simulink model "power_upfc"  (Simulink 8.3)
settings: Solver=ode23tb  SolverMode=SingleTasking  StartTime=0  StopTime=20  MaxStep=1/60  RelTol=1e-4  AbsTol=1e-3
undefined symbols (not defined in the file or in its folder): D1, Delta
libraries: powerlib x30, powerlib_meascontrol x12, sps_avr x2, factslib x1, simulink x1
Description:
  | Copyright 2008-2014 The MathWorks, Inc.
settings Model: Creator=MathWorks  LastModifiedBy=snt  ExtModeAutoUpdateStatusClock=off
settings SolverCC: SolverJacobianMethodControl=FullPerturbation
settings DataIOCC: LimitDataPoints=off  SaveOutput=off  SaveTime=off  SignalLoggingName=sigsOut
settings OptimizationCC: BooleanDataType=off  ExpressionDepthLimit=2147483647  InitFltsAndDblsToZero=on  EfficientMapNaN2IntZero=off
settings DebuggingCC: CheckExecutionContextPreStartOutputMsg=on  CheckExecutionContextRuntimeOutputMsg=on  SignalResolutionControl=TryResolveAllWithWarning  SolverPrmCheckMsg=none  MultiTaskDSMMsg=warning  MultiTaskCondExecSysMsg=none  SigSpecEnsureSampleTimeMsg=none  FcnCallInpInsideContextMsg=UseLocalSettings  UnconnectedInputMsg=none  UnconnectedOutputMsg=none  UnconnectedLineMsg=none
settings HardwareCC: TargetUnknown=on
settings RTWCC: IncludeERTFirstTime=on
settings CodeAppCC: IgnoreCustomStorageClasses=off

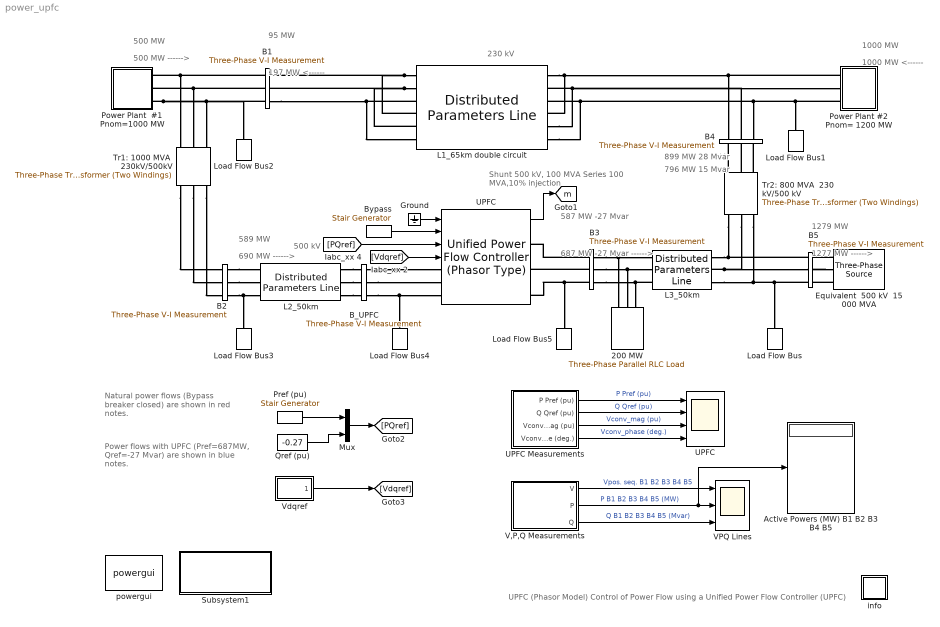
== system power_upfc ==
  note: Shunt 500 kV, 100 MVA
      | Series 100 MVA,10% injection
  note: 1000 MW
      | <------
  note: I
      | I
      | V
  note: 197 MW
      | <------
  note: 1277 MW
      | ------>
  note: 500 MW
      | ------>
  note: 690 MW
      | ------>
  note: 687 MW -27 Mvar
      |           ------>
  note: 230 kV
  note: 500 kV
  note: UPFC (Phasor Model)
      | Control of Power Flow using a Unified Power Flow Controller (UPFC)
  note: 796 MW 15 Mvar
  note: 95 MW
  note: 500 MW
  note: 1000 MW
  note: 589 MW
  note: 587 MW -27 Mvar
  note: 1279 MW
  note: 899 MW 28 Mvar
  note: Natural power flows
      | (Bypass breaker closed)
      | are shown in red notes.
  note: Power flows with UPFC
      | (Pref=687MW, Qref=-27 Mvar)
      | are shown in blue notes.
  200 MW : powerlib/Elements/Three-Phase Parallel RLC Load  LConnTagsString=A|B|C  Configuration=Y (grounded)  NominalVoltage=500e3  NominalFrequency=60  ActivePower=2e+008  InductivePower=0  CapacitivePower=0  Measurements=None  LoadType=constant Z
  Active Powers (MW) B1 B2 B3 B4 B5 : Display
      settings: SampleTime=0.1
  B1 : powerlib/Measurements/Three-Phase V-I Measurement  VoltageMeasurement=phase-to-ground  SetLabelV=on  LabelV=Vabc_B1  Vpu=on  VpuLL=off  CurrentMeasurement=yes  SetLabelI=on  LabelI=Iabc_B1  Ipu=on  Pbase=100e6  Vbase=230e3  OutputType=Complex  PhasorSimulation=on  PSBequivalent=0
  B2 : powerlib/Measurements/Three-Phase V-I Measurement  VoltageMeasurement=phase-to-ground  SetLabelV=on  LabelV=Vabc_B2  Vpu=on  VpuLL=off  CurrentMeasurement=yes  SetLabelI=on  LabelI=Iabc_B2  Ipu=on  Pbase=100e6  Vbase=500e3  OutputType=Complex  PhasorSimulation=on  PSBequivalent=0
  B3 : powerlib/Measurements/Three-Phase V-I Measurement  VoltageMeasurement=phase-to-ground  SetLabelV=on  LabelV=Vabc_B3  Vpu=on  VpuLL=off  CurrentMeasurement=yes  SetLabelI=on  LabelI=Iabc_B3  Ipu=on  Pbase=100e6  Vbase=500e3  OutputType=Complex  PhasorSimulation=on  PSBequivalent=0
  B4 : powerlib/Measurements/Three-Phase V-I Measurement  VoltageMeasurement=phase-to-ground  SetLabelV=on  LabelV=Vabc_B4  Vpu=on  VpuLL=off  CurrentMeasurement=yes  SetLabelI=on  LabelI=Iabc_B4  Ipu=on  Pbase=100e6  Vbase=230e3  OutputType=Complex  PhasorSimulation=on  PSBequivalent=0
  B5 : powerlib/Measurements/Three-Phase V-I Measurement  VoltageMeasurement=phase-to-ground  SetLabelV=on  LabelV=Vabc_B5  Vpu=on  VpuLL=off  CurrentMeasurement=yes  SetLabelI=on  LabelI=Iabc_B5  Ipu=on  Pbase=100e6  Vbase=500e3  OutputType=Complex  PhasorSimulation=on  PSBequivalent=0
  B_UPFC : powerlib/Measurements/Three-Phase V-I Measurement  VoltageMeasurement=phase-to-ground  SetLabelV=on  LabelV=Vabc_UPFC  Vpu=on  VpuLL=off  CurrentMeasurement=no  SetLabelI=on  LabelI=Iabc_UPFC  Ipu=on  Pbase=100e6  Vbase=500e3  OutputType=Complex  PhasorSimulation=on  PSBequivalent=0
  Bypass : powerlib_meascontrol/Pulse & Signal Generators/Stair Generator  t=[0,5]  e=[1, 0]  Ts=0
  Equivalent  500 kV  15 000 MVA : powerlib/Electrical Sources/Three-Phase Source  Voltage=(500000)*1  PhaseAngle=3.2028e-005  Frequency=60  InternalConnection=Yg  SpecifyImpedance=on  Resistance=0.8929  Inductance=16.58e-3  ShortCircuitLevel=15000e6  BaseVoltage=500e3  XRratio=10  BusType=swing  Pref=0  Qref=0  Qmin=-Inf  Qmax=Inf
  Ground : Ground
  L1_65km double circuit : powerlib/Elements/Distributed Parameters Line  Phases=6  Frequency=60  Resistance="[0.068  0.284  0.216]"  Inductance="[1.31e-3  4.02e-3  2.43e-3]"  Capacitance="[8.85e-9  6.21e-9  -1.88e-9]"  Length=65  x1=[1.04987199469285e-07 0 229205.80796604 229205.606293905 229205.80796604 229205.606293905;376.991118430775 376.991118430775 376.991118430775 376.991118430775 376.991118430775 376.991118430775;1.60854183298652 0 0.666699049272692 -0.904097686354923 0.666699049272692 -0.904097686354923]  x2=[6.52522329341896e-07 7.27595761418343e-12 228285.721081789 228285.608536952 228285.721081789 228285.608536952;376.991118430775 376.991118430775 376.991118430775 376.991118430775 376.991118430775 376.991118430775;1.99334329783026 -0.0878855142633377 0.697028223829494 -0.873768326941681 0.697028223829494 -0.873768326941681]  x3=[3.46977339890718e-09 9.30248222866475e-13 797.813028086103 797.813944366895 797.813028086104 797.813944366895;376.991118430775 376.991118430775 376.991118430775 376.991118430775 376.991118430775 376.991118430775;0.713863028790556 0.253093439233012 0.71113154759669 -0.859668364592689 0.71113154759669 -0.859668364592689]  x4=[3.27711624608603e-09 8.10443810681981e-13 388.164983704915 388.162721923639 388.164983704915 388.16272192364;376.991118430775 376.991118430775 376.991118430775 376.991118430775 376.991118430775 376.991118430775;-2.59754346741824 0.0169914244668962 0.493384723437739 -1.07740616674268 0.493384723437737 -1.07740616674268]  x5=0.000343508242259192  V1=ones(3,3)  V2=ones(3,3)  I1=ones(3,3)  I2=ones(3,3)  nHarmo=1  Measurements=None
      settings: AttributesFormatString=\n
  L2_50km : powerlib/Elements/Distributed Parameters Line  Phases=3  Frequency=60  Resistance=[0.01273*2 0.3864]  Inductance="[0.9337e-3  4.1264e-3]"  Capacitance=[12.74e-9 7.751e-9]  Length=50  x1=[5.20853276713395e-08 499627.087562911 499626.799727799;376.991118430775 376.991118430775 376.991118430775;1.55035171690532 0.613862513789087 -0.956934116072279]  x2=[4.53565246682871e-08 499734.367587277 499734.166072354;376.991118430775 376.991118430775 376.991118430775;0.508276734166516 0.572208220004921 -0.998588334903276]  x3=[5.37095681221166e-10 675.32888932722 675.331629163871;376.991118430775 376.991118430775 376.991118430775;-2.03735480978532 0.425693420201668 -1.14510959351009]  x4=[6.51364168678501e-10 3011.82389463488 3011.82010569616;376.991118430775 376.991118430775 376.991118430775;1.09280353932366 0.590627024477705 -0.980167982447582]  x5=0.000282770783497871  V1=ones(3,3)  V2=ones(3,3)  I1=ones(3,3)  I2=ones(3,3)  nHarmo=1  Measurements=None
      settings: AttributesFormatString=\n
  L3_50km : powerlib/Elements/Distributed Parameters Line  Phases=3  Frequency=60  Resistance=[0.01273*2 0.3864]  Inductance="[0.9337e-3  4.1264e-3]"  Capacitance=[12.74e-9 7.751e-9]  Length=50  x1=[4.54922196369805e-08 499734.250125523 499734.048610914;376.991118430775 376.991118430775 376.991118430775;0.506954071581508 0.572208208878681 -0.998588346030441]  x2=[7.60694684117164e-08 498857.669479026 498857.551895537;376.991118430775 376.991118430775 376.991118430775;-0.0702475012256047 0.544899092106288 -1.02589737598285]  x3=[5.13234018676451e-10 1067.88465961171 1067.8871249624;376.991118430775 376.991118430775 376.991118430775;-1.90562270617231 0.520240004579847 -1.0505607358324]  x4=[5.95962577824804e-10 2609.42085232127 2609.41725096603;376.991118430775 376.991118430775 376.991118430775;0.999199616559189 0.528387817683497 -1.04240695612209]  x5=0.000282770783497871  V1=ones(3,3)  V2=ones(3,3)  I1=ones(3,3)  I2=ones(3,3)  nHarmo=1  Measurements=None
      settings: AttributesFormatString=\n
  Load Flow Bus : powerlib/Measurements/Load Flow Bus  LConnTagsString=a  ID=B5  Vbase=500e3  Vref=0.997715  Vangle=4.9453  VLF=0.9977  angleLF=4.945
      settings: AttributesFormatString=%<ID>\n%<Vbase>V\n%<VLF>pu\n%<angleLF>deg.
  Load Flow Bus1 : powerlib/Measurements/Load Flow Bus  LConnTagsString=a  ID=B4  Vbase=230e3  Vref=1  Vangle=0  VLF=0.9925  angleLF=14.72
      settings: AttributesFormatString=%<ID>\n%<Vbase>V\n%<VLF>pu\n%<angleLF>deg.
  Load Flow Bus2 : powerlib/Measurements/Load Flow Bus  LConnTagsString=a  ID=B1  Vbase=230e3  Vref=1  Vangle=0  VLF=0.9965  angleLF=12.98
      settings: AttributesFormatString=%<ID>\n%<Vbase>V\n%<VLF>pu\n%<angleLF>deg.
  Load Flow Bus3 : powerlib/Measurements/Load Flow Bus  LConnTagsString=a  ID=B2  Vbase=500e3  Vref=1  Vangle=0  VLF=0.9993  angleLF=8.897
      settings: AttributesFormatString=%<ID>\n%<Vbase>V\n%<VLF>pu\n%<angleLF>deg.
  Load Flow Bus4 : powerlib/Measurements/Load Flow Bus  LConnTagsString=a  ID=B_UPFC  Vbase=500e3  Vref=1  Vangle=0  VLF=0.9995  angleLF=6.51
      settings: AttributesFormatString=%<ID>\n%<Vbase>V\n%<VLF>pu\n%<angleLF>deg.
  Load Flow Bus5 : powerlib/Measurements/Load Flow Bus  LConnTagsString=a  ID=B3  Vbase=500e3  Vref=1  Vangle=0  VLF=0.9995  angleLF=6.51
      settings: AttributesFormatString=%<ID>\n%<Vbase>V\n%<VLF>pu\n%<angleLF>deg.
  Mux : Mux  Inputs=2
  Power Plant  #1 Pnom=1000 MW : Subsystem
  Power Plant #2 Pnom= 1200 MW : Subsystem
  Pref (pu) : powerlib_meascontrol/Pulse & Signal Generators/Stair Generator  t=[0,10]  e="[5.87 6.87  ]"  Ts=0
  Qref (pu) : Constant  Value=-0.27
  Subsystem1 : Subsystem
      settings: OpenFcn=|
      | if exist('P_SE') & exist('Q_SE')
      | plot(P_SE(300:length(Q_SE),2),Q_SE(300:length(Q_SE),2))
      | pbaspect([1 1 1]);
      |    grid
      | title('UPFC Controllable Region')
      | xlabel ('P (pu)')
      | ylabel ('Q (pu)')
      | end
      mask Display: disp('Double click to plot\nUPFC\nControllable Region')
  Tr1: 1000 MVA  230kV/500kV : powerlib/Elements/Three-Phase Transformer (Two Windings)  Winding1Connection=Yg  UNITS=pu  NominalPower=[ 1000e6 60 ]  Winding1="[ 230e3 0.002  0.0]"  Winding2Connection=Yg  Winding2=[ 500e3 0.002 0.12]  SetSaturation=off  Rm=500  Lm=500  Saturation="[ 0,0  ;  0.005,1.2  ;  1.0,1.4 ]"  Hysteresis=off  DataFile='basic_model'  SetInitialFlux=off  InitialFluxes=[ 0.8 , -0.8 , 0.7 ]  Measurements=None  MoreParameters=off  BreakLoop=off  DataType=off  TransfoNumber=0
  Tr2: 800 MVA  230 kV/500 kV : powerlib/Elements/Three-Phase Transformer (Two Windings)  Winding1Connection=Yg  UNITS=pu  NominalPower=[ 800e6 60 ]  Winding1="[ 230e3 0.002  0.0]"  Winding2Connection=Yg  Winding2=[ 500e3 0.002 0.15]  SetSaturation=off  Rm=500  Lm=500  Saturation="[ 0,0  ;  0.005,1.2  ;  1.0,1.4 ]"  Hysteresis=off  DataFile='basic_model'  SetInitialFlux=off  InitialFluxes=[ 0.8 , -0.8 , 0.7 ]  Measurements=None  MoreParameters=off  BreakLoop=off  DataType=off  TransfoNumber=0
  UPFC : factslib/Power-Electronics Based FACTS/Unified Power Flow Controller (Phasor Type)  ShowParameters=Control parameters (series converter)  SystemNominal=[ 500e3, 60 ]  Pnom_SH=100e6  RL_SH=[ 0.22/30, 0.22 ]  Iinit_SH=[0, 0 ]  SeriesNominal=[ 100e6, 0.1]  RL_SE=[ 0.16/30, 0.16 ]  Iinit_SE=[ 0 0]  VnomDC=40000  C_DC=750e-6  OpMode_SH=Voltage regulation  ExternalVref=off  Vref_SH=1.00  MaxRateChangeVref_SH=0.1  Droop_SH=0.03  Par_VacReg=[5 1000]  Qref_SH=0  MaxRateChangeQref_SH=2  Par_VdcReg=[0.1e-3 20e-3]  Par_IReg_SH=[0.5 25]/3  ExternalByPass=External control  OpMode_SE=Power flow control  ExternalPQref=on  PQref_SE=[5.87 -0.27]  Rate_PQref=1  Par_PReg_SE=[0.025 1.5]  ExternalVdqref=on  Vdqref_SE=[0.05 0.05]  Rate_Vdqref=0.2
  UPFC Measurements : Subsystem
      mask Display: disp('UPFC\nMeasurements')
  "UPFC " : Scope  NumInputPorts=4
      settings: TimeRange=20  YMin=5.5~-0.29~0~90  YMax=7~-0.26~0.1~96
  V,P,Q Measurements : Subsystem
      mask Display: disp('V P Q\nMeasurements')
  VPQ Lines : Scope  NumInputPorts=3
      settings: TimeRange=20  YMin=0.99~0~-150  YMax=1.005~1500~50
  Vdqref : Subsystem
  info : Subsystem
      settings: OpenFcn=showdemo(bdroot(gcb))
      mask Display: disp('?')
  powergui : powerlib/powergui  Priority=2  SimulationMode=Phasor  SolverType=Tustin  SampleTime=0  frequency=60  SPID=off  DisableSnubberDevices=off  DisableRonSwitches=off  DisableVfSwitches=off  SwTol=0  Interpol=off  DisplayEquations=off  Ts=0  methode=off  frequencyindice=60  Pbase=100e6  ErrMax=0.0001  Iterations=50  UnitsV=kV  UnitsW=MW  FunctionMessages=off  echomessages=off  HookPort=off  EnableUseOfTLC=off  x0status=blocks  RestoreLinks=warning  ResistiveCurrentMeasurement=off  Frange=[0:2:500]  Ylog=off  Xlog=off  ShowGrid=off  save=off  variable=ZData  structure=0  ZoomFFT=on  StartTime=0.0  cycles=1  DisplayStyle=off  fundamental=60  FreqAxis=off  MaxFrequency=1000  frequencyindicesteady=1  RmsSteady=2  display=off
  tag scope: m=global
  wires:
  Pref (pu)/1 -> Mux/1
  Qref (pu)/1 -> Mux/2
  Mux/1 -> [PQref]
  V,P,Q Measurements/1(V) -> VPQ Lines/1  "Vpos. seq. B1 B2 B3 B4 B5"
  UPFC/1 -> [m]
  Vdqref/1(Vdqref) -> [Vdqref]
  V,P,Q Measurements/3(Q) -> VPQ Lines/3  "Q B1 B2 B3 B4 B5 (Mvar)"
  UPFC Measurements/1(P Pref (pu)) -> "UPFC "/1  "P Pref (pu)"
  UPFC Measurements/2(Q Qref (pu)) -> "UPFC "/2  "Q Qref (pu)"
  UPFC Measurements/3(Vconv_mag (pu)) -> "UPFC "/3  "Vconv_mag (pu)"
  UPFC Measurements/4(Vconv_phase (deg.)) -> "UPFC "/4  "Vconv_phase (deg.)"
  V,P,Q Measurements/2(P) -> VPQ Lines/2, Active Powers (MW) B1 B2 B3 B4 B5/1  "P B1 B2 B3 B4 B5 (MW)"
  Ground/1 -> UPFC/1
  [Vdqref] -> UPFC/4
  [PQref] -> UPFC/3
  Bypass/1 -> UPFC/2
  connections:
  Equivalent  500 kV  15 000 MVA/RConn1 -- B5/RConn1
  B5/RConn2 -- Equivalent  500 kV  15 000 MVA/RConn2
  Equivalent  500 kV  15 000 MVA/RConn3 -- B5/RConn3
  Power Plant #2 Pnom= 1200 MW/RConn3 -- L1_65km double circuit/RConn3 -- L1_65km double circuit/RConn6 -- B4/LConn3 -- Load Flow Bus1/LConn1
  L3_50km/RConn1 -- B5/LConn1 -- Tr2: 800 MVA  230 kV/500 kV/RConn1
  L3_50km/RConn2 -- B5/LConn2 -- Tr2: 800 MVA  230 kV/500 kV/RConn2
  B5/LConn3 -- L3_50km/RConn3 -- Tr2: 800 MVA  230 kV/500 kV/RConn3 -- Load Flow Bus/LConn1
  B4/LConn2 -- Power Plant #2 Pnom= 1200 MW/RConn2 -- L1_65km double circuit/RConn2 -- L1_65km double circuit/RConn5
  B3/RConn1 -- L3_50km/LConn1 -- 200 MW/LConn1
  B3/RConn2 -- L3_50km/LConn2 -- 200 MW/LConn2
  B3/RConn3 -- L3_50km/LConn3 -- 200 MW/LConn3
  B2/RConn1 -- L2_50km/LConn1
  B2/RConn2 -- L2_50km/LConn2
  B2/RConn3 -- L2_50km/LConn3 -- Load Flow Bus3/LConn1
  B1/RConn1 -- Power Plant  #1 Pnom=1000 MW/RConn1 -- Tr1: 1000 MVA  230kV/500kV/LConn1
  B1/RConn2 -- Power Plant  #1 Pnom=1000 MW/RConn2 -- Tr1: 1000 MVA  230kV/500kV/LConn2
  Power Plant  #1 Pnom=1000 MW/RConn3 -- B1/RConn3 -- Load Flow Bus2/LConn1 -- Tr1: 1000 MVA  230kV/500kV/LConn3
  Tr1: 1000 MVA  230kV/500kV/RConn1 -- B2/LConn1
  Tr1: 1000 MVA  230kV/500kV/RConn2 -- B2/LConn2
  Tr1: 1000 MVA  230kV/500kV/RConn3 -- B2/LConn3
  Tr2: 800 MVA  230 kV/500 kV/LConn1 -- B4/RConn1
  Tr2: 800 MVA  230 kV/500 kV/LConn2 -- B4/RConn2
  Tr2: 800 MVA  230 kV/500 kV/LConn3 -- B4/RConn3
  L2_50km/RConn1 -- B_UPFC/LConn1
  L2_50km/RConn2 -- B_UPFC/LConn2
  L2_50km/RConn3 -- B_UPFC/LConn3
  B_UPFC/RConn1 -- UPFC/LConn1
  B_UPFC/RConn2 -- UPFC/LConn2
  B_UPFC/RConn3 -- UPFC/LConn3 -- Load Flow Bus4/LConn1
  B3/LConn1 -- UPFC/RConn1
  B3/LConn2 -- UPFC/RConn2
  B3/LConn3 -- UPFC/RConn3 -- Load Flow Bus5/LConn1
  L1_65km double circuit/LConn1 -- B1/LConn1 -- L1_65km double circuit/LConn4
  L1_65km double circuit/LConn2 -- B1/LConn2 -- L1_65km double circuit/LConn5
  B1/LConn3 -- L1_65km double circuit/LConn3 -- L1_65km double circuit/LConn6
  L1_65km double circuit/RConn1 -- Power Plant #2 Pnom= 1200 MW/RConn1 -- B4/LConn1 -- L1_65km double circuit/RConn4

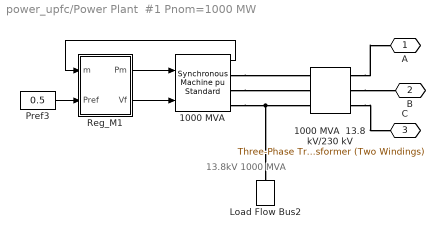
== system power_upfc/Power Plant  #1 Pnom=1000 MW ==
  note: 13.8kV 1000 MVA
  1000 MVA : powerlib/Machines/Synchronous Machine pu Standard  PresetModel=No  MechanicalLoad=Mechanical power Pm  ShowDetailedParameters=on  RotorType=Salient-pole  Units=per unit standard parameters  MeasurementBus=off  NominalParameters="[1000E6  13800   60 ]"  Reactances1=[ 31 32 33 34 35 36 37 ]  Reactances2=[ 1.305, 0.296, 0.252, 0.474, 0.243, 0.18 ]  dAxisTimeConstants=Short-circuit  qAxisTimeConstants=Open-circuit  TimeConstants1=[]  TimeConstants2=[]  TimeConstants3=[]  TimeConstants4=[]  TimeConstants5=[ 1.01, 0.053, 0.1 ]  TimeConstants6=[]  TimeConstants7=[]  TimeConstants8=[]  StatorResistance=2.8544e-3  Mechanical="[ 3.7 0  32]"  PolePairs=32  InitialConditions=[0 -90.4528 0.500842 0.500842 0.500842 -16.9126 -136.913 103.087 1.1604]  SetSaturation=off  Saturation=[0.6404,0.7127,0.8441,0.9214,0.9956,1.082,1.19,1.316,1.457;0.7,0.7698,0.8872,0.9466,0.9969,1.046,1.1,1.151,1.201]  LoadFlowParameters=[1 500000000 0 0 0]  TsPowergui=0  TsBlock=-1  IterativeModel=Forward Euler  BusType=PV  Pref=5e+008  Qref=0  Qmin=-Inf  Qmax=Inf  PLF=0  QLF=0
      settings: AttributesFormatString=\n\n
  1000 MVA  13.8 kV/230 kV : powerlib/Elements/Three-Phase Transformer (Two Windings)  Winding1Connection=Delta (D1)  UNITS=pu  NominalPower=[ 1000e6 60 ]  Winding1="[ 13.8e3 0.002  0.0]"  Winding2Connection=Yg  Winding2=[ 230e3 0.002 0.12]  SetSaturation=off  Rm=500  Lm=500  Saturation="[ 0,0  ;  0.005,1.2  ;  1.0,1.4 ]"  Hysteresis=off  DataFile='basic_model'  SetInitialFlux=off  InitialFluxes=[ 0.8 , -0.8 , 0.7 ]  Measurements=None  MoreParameters=off  BreakLoop=off  DataType=off  TransfoNumber=0
  Load Flow Bus2 : powerlib/Measurements/Load Flow Bus  LConnTagsString=a  ID=M1  Vbase=13.8e3  Vref=1  Vangle=0  VLF=1  angleLF=-13.59
      settings: AttributesFormatString=%<ID>\n%<Vbase>V\n%<VLF>pu\n%<angleLF>deg.
  Pref3 : Constant  Value=0.5
  Reg_M1 : Subsystem
  A : PMIOPort  Port=1  Side=Right
  B : PMIOPort  Port=2  Side=Right
  C : PMIOPort  Port=3  Side=Right
  wires:
  Reg_M1/1(Pm) -> 1000 MVA/1
  Reg_M1/2(Vf) -> 1000 MVA/2
  Pref3/1 -> Reg_M1/2(Pref)
  1000 MVA/1 -> Reg_M1/1(m)
  connections:
  1000 MVA/RConn1 -- 1000 MVA  13.8 kV/230 kV/LConn1
  1000 MVA/RConn2 -- 1000 MVA  13.8 kV/230 kV/LConn2
  1000 MVA/RConn3 -- 1000 MVA  13.8 kV/230 kV/LConn3 -- Load Flow Bus2/LConn1
  1000 MVA  13.8 kV/230 kV/RConn1 -- A/RConn1
  1000 MVA  13.8 kV/230 kV/RConn2 -- B/RConn1
  1000 MVA  13.8 kV/230 kV/RConn3 -- C/RConn1

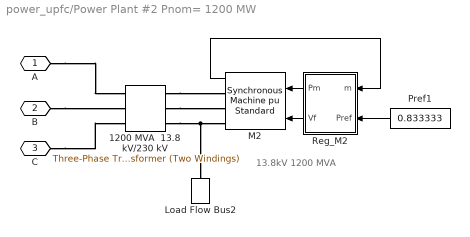
== system power_upfc/Power Plant #2 Pnom= 1200 MW ==
  note: 13.8kV 1200 MVA
  1200 MVA  13.8 kV/230 kV : powerlib/Elements/Three-Phase Transformer (Two Windings)  Winding1Connection=Delta (D1)  UNITS=pu  NominalPower=[ 1200e6 60 ]  Winding1="[ 13.8e3 0.002  0.0]"  Winding2Connection=Yg  Winding2=[ 230e3 0.002 0.12]  SetSaturation=off  Rm=500  Lm=500  Saturation="[ 0,0  ;  0.005,1.2  ;  1.0,1.4 ]"  Hysteresis=off  DataFile='basic_model'  SetInitialFlux=off  InitialFluxes=[ 0.8 , -0.8 , 0.7 ]  Measurements=None  MoreParameters=off  BreakLoop=off  DataType=off  TransfoNumber=0
  Load Flow Bus2 : powerlib/Measurements/Load Flow Bus  LConnTagsString=a  ID=M2  Vbase=13.8e3  Vref=1  Vangle=0  VLF=1  angleLF=-9.532
      settings: AttributesFormatString=%<ID>\n%<Vbase>V\n%<VLF>pu\n%<angleLF>deg.
  M2 : powerlib/Machines/Synchronous Machine pu Standard  PresetModel=No  MechanicalLoad=Mechanical power Pm  ShowDetailedParameters=on  RotorType=Salient-pole  Units=per unit standard parameters  MeasurementBus=off  NominalParameters="[1200E6  13800   60 ]"  Reactances1=[ 31 32 33 34 35 36 37 ]  Reactances2=[ 1.305, 0.296, 0.252, 0.474, 0.243, 0.18 ]  dAxisTimeConstants=Short-circuit  qAxisTimeConstants=Open-circuit  TimeConstants1=[]  TimeConstants2=[]  TimeConstants3=[]  TimeConstants4=[]  TimeConstants5=[ 1.01, 0.053, 0.1 ]  TimeConstants6=[]  TimeConstants7=[]  TimeConstants8=[]  StatorResistance=2.8544e-3  Mechanical="[ 3.7 0  32]"  PolePairs=32  InitialConditions=[0 -78.7337 0.836975 0.836975 0.836975 -14.879 -134.879 105.121 1.41828]  SetSaturation=off  Saturation=[0.6404,0.7127,0.8441,0.9214,0.9956,1.082,1.19,1.316,1.457;0.7,0.7698,0.8872,0.9466,0.9969,1.046,1.1,1.151,1.201]  LoadFlowParameters=[1 1000000000 0 0 0]  TsPowergui=0  TsBlock=-1  IterativeModel=Forward Euler  BusType=PV  Pref=1e+009  Qref=0  Qmin=-Inf  Qmax=Inf  PLF=0  QLF=0
      settings: AttributesFormatString=\n\n
  Pref1 : Constant  Value=0.833333
  Reg_M2 : Subsystem
  A : PMIOPort  Port=1  Side=Right
  B : PMIOPort  Port=2  Side=Right
  C : PMIOPort  Port=3  Side=Right
  wires:
  Reg_M2/1(Pm) -> M2/1
  Reg_M2/2(Vf) -> M2/2
  Pref1/1 -> Reg_M2/2(Pref)
  M2/1 -> Reg_M2/1(m)
  connections:
  1200 MVA  13.8 kV/230 kV/LConn1 -- M2/RConn1
  1200 MVA  13.8 kV/230 kV/LConn2 -- M2/RConn2
  1200 MVA  13.8 kV/230 kV/LConn3 -- M2/RConn3 -- Load Flow Bus2/LConn1
  A/RConn1 -- 1200 MVA  13.8 kV/230 kV/RConn1
  B/RConn1 -- 1200 MVA  13.8 kV/230 kV/RConn2
  C/RConn1 -- 1200 MVA  13.8 kV/230 kV/RConn3

== system power_upfc/Subsystem1 ==

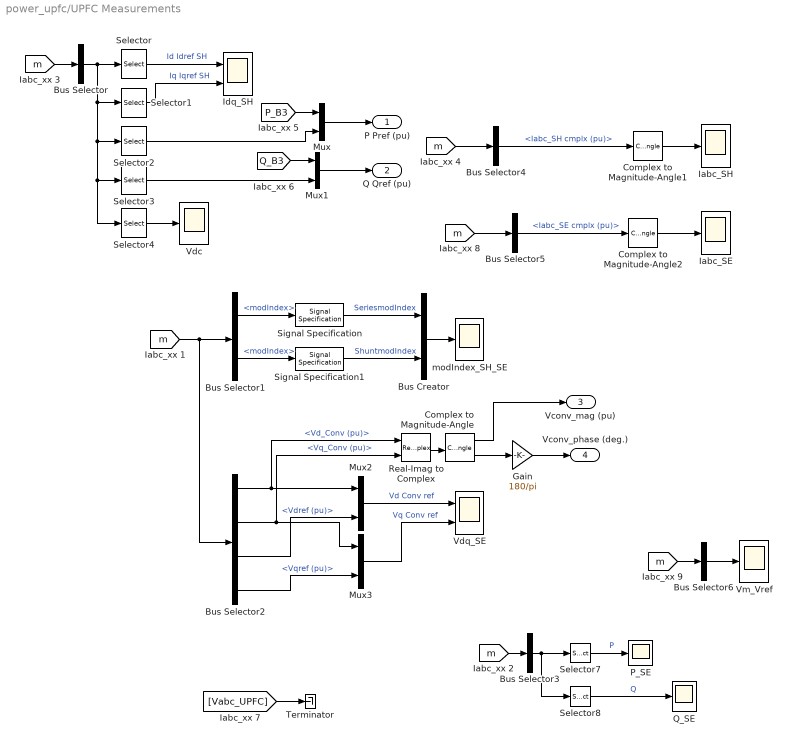
== system power_upfc/UPFC Measurements ==
  Bus Creator : BusCreator  Inputs=2
  Bus Selector : BusSelector  OutputSignals=Control (Shunt).Id (pu),Control (Shunt).Iq (pu),Control (Shunt).Idref (pu),Control (Shunt).Iqref (pu),Control (Series).P (pu),Control (Series).Q (pu),Control (Series).Pref (pu),Control (Series).Qref (pu),Power.Vdc (V)  OutputAsBus=on
  Bus Selector1 : BusSelector  OutputSignals=Control (Shunt).modIndex,Control (Series).modIndex
  Bus Selector2 : BusSelector  OutputSignals=Control (Series).Vd_Conv (pu),Control (Series).Vq_Conv (pu),Control (Series).Vdref (pu),Control (Series).Vqref (pu)
  Bus Selector3 : BusSelector  OutputSignals=Control (Series).P (pu),Control (Series).Pref (pu),Control (Series).Q (pu),Control (Series).Qref (pu)  OutputAsBus=on
  Bus Selector4 : BusSelector  OutputSignals=Power.Iabc_SH cmplx (pu)
  Bus Selector5 : BusSelector  OutputSignals=Power.Iabc_SE cmplx (pu)
  Bus Selector6 : BusSelector  OutputSignals=Control (Shunt).Vm (pu),Control (Shunt).Vref (pu)  OutputAsBus=on
  Complex to Magnitude-Angle : ComplexToMagnitudeAngle
  Complex to Magnitude-Angle1 : ComplexToMagnitudeAngle  Output=Magnitude
  Complex to Magnitude-Angle2 : ComplexToMagnitudeAngle  Output=Magnitude
  Gain : Gain  Gain=180/pi  SaturateOnIntegerOverflow=on  OutDataTypeStr=Inherit: Same as input  ParamDataTypeStr=Inherit: Same as input
  Iabc_SE : Scope
      settings: YMin=4.8  YMax=6.9  SaveName=ScopeData8
  Iabc_SH : Scope
      settings: YMin=0  YMax=0.004  SaveName=ScopeData5
  Idq_SH : Scope  NumInputPorts=2
      settings: YMin=-1~-1  YMax=1~1
  Mux{,1..3} (4 alike) : Mux  Inputs=2
  P_SE : Scope
      settings: YMin=1  YMax=10  SaveName=P_SE  SampleTime=1/60
  Q_SE : Scope
      settings: YMin=1  YMax=10  SaveName=Q_SE  SampleTime=1/60
  Real-Imag to Complex : RealImagToComplex
  Selector : Selector  InputPortWidth=9  Indices=[1 3]
  Selector1 : Selector  InputPortWidth=9  Indices=[1 3]+1
  Selector2 : Selector  InputPortWidth=9  Indices=[7]
  Selector3 : Selector  InputPortWidth=9  Indices=[8]
  Selector4 : Selector  InputPortWidth=9  Indices=9
  Selector7 : Selector  InputPortWidth=4  Indices=[1 2]
  Selector8 : Selector  InputPortWidth=4  Indices=[1 2]+2
  Signal Specification : SignalSpecification
  Signal Specification1 : SignalSpecification
  Terminator : Terminator
  Vdc : Scope
      settings: YMin=38100  YMax=40100  SaveName=ScopeData3
  Vdq_SE : Scope  NumInputPorts=2
      settings: YMin=-0.125~-0.125  YMax=0.125~0.125  SaveName=ScopeData2
  Vm_Vref : Scope
      settings: YMin=0.5  YMax=1.5  SaveName=ScopeData7
  modIndex_SH_SE : Scope
      settings: YMin=0  YMax=0.75  SaveName=ScopeData11
  P Pref (pu) : Outport
  Q Qref (pu) : Outport  Port=2
  Vconv_mag (pu) : Outport  Port=3
  Vconv_phase (deg.) : Outport  Port=4
  wires:
  Mux1/1 -> Q Qref (pu)/1
  Selector3/1 -> Mux1/2
  [m] -> Bus Selector/1
  Selector/1 -> Idq_SH/1  "Id Idref SH"
  Selector1/1 -> Idq_SH/2  "Iq Iqref SH"
  Bus Selector/1 -> Selector/1, Selector1/1, Selector4/1, Selector3/1, Selector2/1
  Selector4/1 -> Vdc/1
  [m] -> Bus Selector2/1, Bus Selector1/1
  [P_B3] -> Mux/1
  [Q_B3] -> Mux1/1
  Selector2/1 -> Mux/2
  Mux2/1 -> Vdq_SE/1  "Vd Conv ref"
  Mux3/1 -> Vdq_SE/2  "Vq Conv ref"
  [m] -> Bus Selector3/1
  Bus Selector3/1 -> Selector7/1, Selector8/1
  Selector7/1 -> P_SE/1  "P"
  Mux/1 -> P Pref (pu)/1
  Selector8/1 -> Q_SE/1  "Q"
  [Vabc_UPFC] -> Terminator/1
  Real-Imag to Complex/1 -> Complex to Magnitude-Angle/1
  Complex to Magnitude-Angle/2 -> Gain/1
  Gain/1 -> Vconv_phase (deg.)/1
  Complex to Magnitude-Angle/1 -> Vconv_mag (pu)/1
  Bus Selector2/1 -> Mux2/1, Real-Imag to Complex/1  "<Vd_Conv (pu)>"
  Bus Selector2/3 -> Mux2/2  "<Vdref (pu)>"
  Bus Selector2/2 -> Mux3/1, Real-Imag to Complex/2  "<Vq_Conv (pu)>"
  Bus Selector2/4 -> Mux3/2  "<Vqref (pu)>"
  [m] -> Bus Selector4/1
  Bus Selector4/1 -> Complex to Magnitude-Angle1/1  "<Iabc_SH cmplx (pu)>"
  Complex to Magnitude-Angle1/1 -> Iabc_SH/1
  [m] -> Bus Selector5/1
  Bus Selector5/1 -> Complex to Magnitude-Angle2/1  "<Iabc_SE cmplx (pu)>"
  Complex to Magnitude-Angle2/1 -> Iabc_SE/1
  [m] -> Bus Selector6/1
  Bus Selector6/1 -> Vm_Vref/1
  Bus Creator/1 -> modIndex_SH_SE/1
  Bus Selector1/1 -> Signal Specification/1  "<modIndex>"
  Signal Specification/1 -> Bus Creator/1  "SeriesmodIndex"
  Bus Selector1/2 -> Signal Specification1/1  "<modIndex>"
  Signal Specification1/1 -> Bus Creator/2  "ShuntmodIndex"

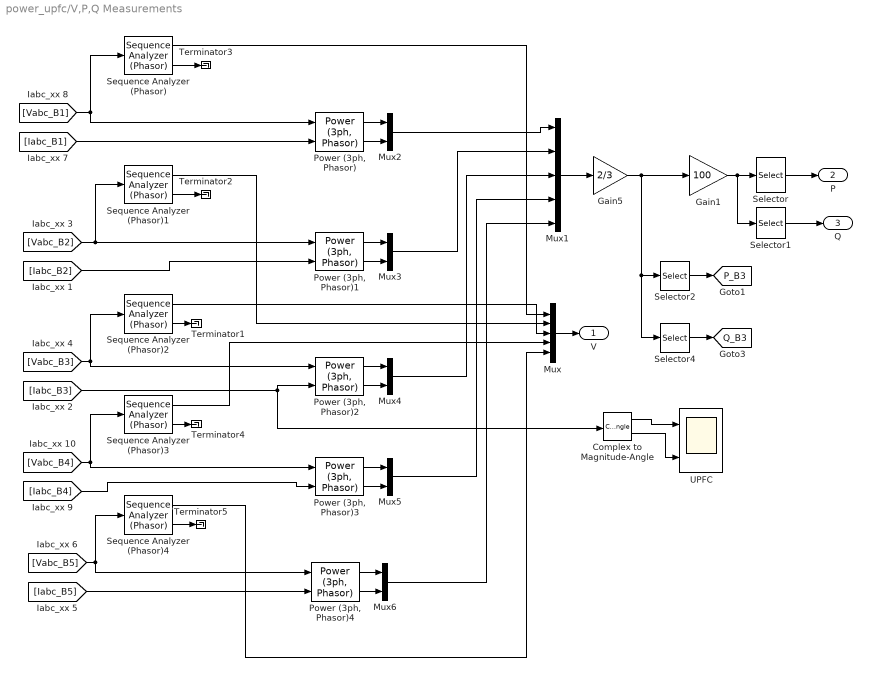
== system power_upfc/V,P,Q Measurements ==
  Complex to Magnitude-Angle : ComplexToMagnitudeAngle
  Gain1 : Gain  Gain=100  SaturateOnIntegerOverflow=on  OutDataTypeStr=Inherit: Same as input  ParamDataTypeStr=Inherit: Same as input
  Gain5 : Gain  Gain=2/3  SaturateOnIntegerOverflow=on  OutDataTypeStr=Inherit: Same as input  ParamDataTypeStr=Inherit: Same as input
  Mux : Mux  Inputs=5
  Mux1 : Mux  Inputs=5
  Mux{2..6} (5 alike) : Mux  Inputs=2
  Power (3ph, Phasor){,1..4} (5 alike) : powerlib_meascontrol/Measurements/Power (3ph, Phasor)
  Selector : Selector  InputPortWidth=10  Indices=[1 3 5 7 9 ]
  Selector1 : Selector  InputPortWidth=10  Indices=[1 3 5 7 9 ]+1
  Selector2 : Selector  InputPortWidth=10  Indices=5
  Selector4 : Selector  InputPortWidth=10  Indices=6
  Sequence Analyzer (Phasor){,1..4} (5 alike) : powerlib_meascontrol/Measurements/Sequence Analyzer (Phasor)  seq=Positive
  Terminator{1..5} (5 alike) : Terminator
  "UPFC " : Scope  NumInputPorts=2
      settings: YMin=5.5~-1.25  YMax=8~1.5  SaveName=ScopeData6
  V : Outport
  P : Outport  Port=2
  Q : Outport  Port=3
  tag scope: P_B3=global, Q_B3=global
  wires:
  Sequence Analyzer (Phasor)4/2 -> Terminator5/1
  Sequence Analyzer (Phasor)/1 -> Mux/1
  Sequence Analyzer (Phasor)3/1 -> Mux/4
  Sequence Analyzer (Phasor)4/1 -> Mux/5
  Mux6/1 -> Mux1/5
  Mux2/1 -> Mux1/1
  Mux5/1 -> Mux1/4
  Sequence Analyzer (Phasor)3/2 -> Terminator4/1
  [Iabc_B4] -> "Power (3ph, Phasor)3"/2
  [Vabc_B4] -> Sequence Analyzer (Phasor)3/1, "Power (3ph, Phasor)3"/1
  [Iabc_B1] -> "Power (3ph, Phasor)"/2
  [Vabc_B1] -> "Power (3ph, Phasor)"/1, Sequence Analyzer (Phasor)/1
  Selector1/1 -> Q/1
  Selector/1 -> P/1
  Mux1/1 -> Gain5/1
  Mux/1 -> V/1
  Mux4/1 -> Mux1/3
  Mux3/1 -> Mux1/2
  Sequence Analyzer (Phasor)2/1 -> Mux/3
  Sequence Analyzer (Phasor)1/1 -> Mux/2
  Sequence Analyzer (Phasor)2/2 -> Terminator1/1
  [Iabc_B5] -> "Power (3ph, Phasor)4"/2
  [Vabc_B5] -> "Power (3ph, Phasor)4"/1, Sequence Analyzer (Phasor)4/1
  [Iabc_B3] -> "Power (3ph, Phasor)2"/2, Complex to Magnitude-Angle/1
  [Vabc_B3] -> "Power (3ph, Phasor)2"/1, Sequence Analyzer (Phasor)2/1
  [Iabc_B2] -> "Power (3ph, Phasor)1"/2
  [Vabc_B2] -> "Power (3ph, Phasor)1"/1, Sequence Analyzer (Phasor)1/1
  Sequence Analyzer (Phasor)1/2 -> Terminator2/1
  Gain5/1 -> Gain1/1, Selector2/1, Selector4/1
  Selector2/1 -> [P_B3]
  Gain1/1 -> Selector1/1, Selector/1
  Selector4/1 -> [Q_B3]
  Sequence Analyzer (Phasor)/2 -> Terminator3/1
  Complex to Magnitude-Angle/1 -> "UPFC "/1
  Complex to Magnitude-Angle/2 -> "UPFC "/2
  "Power (3ph, Phasor)"/2 -> Mux2/2
  "Power (3ph, Phasor)"/1 -> Mux2/1
  "Power (3ph, Phasor)1"/2 -> Mux3/2
  "Power (3ph, Phasor)1"/1 -> Mux3/1
  "Power (3ph, Phasor)2"/2 -> Mux4/2
  "Power (3ph, Phasor)2"/1 -> Mux4/1
  "Power (3ph, Phasor)3"/2 -> Mux5/2
  "Power (3ph, Phasor)3"/1 -> Mux5/1
  "Power (3ph, Phasor)4"/2 -> Mux6/2
  "Power (3ph, Phasor)4"/1 -> Mux6/1

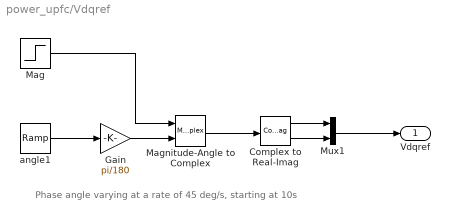
== system power_upfc/Vdqref ==
  note: Phase angle varying at a rate of 45 deg/s, starting at 10s
  Complex to Real-Imag : ComplexToRealImag
  Gain : Gain  Gain=pi/180  SaturateOnIntegerOverflow=on  OutDataTypeStr=Inherit: Same as input  ParamDataTypeStr=Inherit: Same as input
  Mag : Step  Time=5  Before=0.0094  After=0.1  SampleTime=0
  Magnitude-Angle to Complex : MagnitudeAngleToComplex
  Mux1 : Mux  Inputs=2
  angle1 : simulink/Sources/Ramp  slope=90/2  start=10  X0=90.75
  Vdqref : Outport
  wires:
  Gain/1 -> Magnitude-Angle to Complex/2
  Magnitude-Angle to Complex/1 -> Complex to Real-Imag/1
  Complex to Real-Imag/1 -> Mux1/1
  Complex to Real-Imag/2 -> Mux1/2
  angle1/1 -> Gain/1
  Mux1/1 -> Vdqref/1
  Mag/1 -> Magnitude-Angle to Complex/1

== system power_upfc/info ==

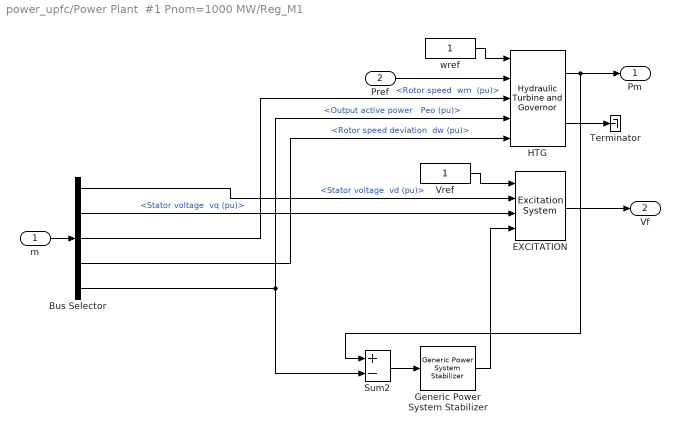
== system power_upfc/Power Plant  #1 Pnom=1000 MW/Reg_M1 ==
  m : Inport
  Pref : Inport  Port=2
  Bus Selector : BusSelector  OutputSignals="dq0 components.Stator voltage  vd (pu),dq0 components.Stator voltage  vq (pu),Mechanical.Rotor speed  wm  (pu),Mechanical.Rotor speed deviation  dw (pu),Output active power   Peo (pu)"
  EXCITATION : sps_avr/Excitation System  tr=20e-3  reg=[ 200, 0.001 ]  exc=[ 1, 0 ]  tgr=[ 0, 0 ]  damp=[ 0.001, 0.1 ]  sat=[ 0, 0 ]  lim="[ 0,  7, 0 ]"  v0=[1,1.1604]
  Generic Power System Stabilizer : powerlib/Machines/Generic Power System Stabilizer  Tsensor=15e-3  K=2.5  Twashout=1  Tleadlag1="[0.06  1]"  Tleadlag2="[0  0]"  VSlimits=[-0.15 0.15]  Vinit=0  Plot_On=off  MagdB_On=on  FreqRange=logspace(-2,2,500)
  HTG : powerlib/Machines/Hydraulic Turbine and Governor  sm="[ 10/3  0.07 ]"  gate="[  0.01  0.97518  -0.1  0.1 ]"  reg="[  0.05  1.163  0.105  0  0.01  ]"  hyd="[  0  2.67  ]"  dref=0  po=0.500716
  Sum2 : Sum  Inputs=+-  SaturateOnIntegerOverflow=on  InputSameDT=on  OutDataTypeStr=Inherit: Same as first input
  Terminator : Terminator
  Vref : Constant
  wref : Constant
  Pm : Outport  InitialOutput=0
  Vf : Outport  Port=2  InitialOutput=0
  wires:
  HTG/2 -> Terminator/1
  Vref/1 -> EXCITATION/1
  m/1 -> Bus Selector/1
  Bus Selector/4 -> HTG/5  "<Rotor speed deviation  dw (pu)>"
  Bus Selector/5 -> HTG/4, Sum2/2  "<Output active power   Peo (pu)>"
  Bus Selector/3 -> HTG/3  "<Rotor speed  wm  (pu)>"
  Pref/1 -> HTG/2
  wref/1 -> HTG/1
  HTG/1 -> Pm/1, Sum2/1
  Bus Selector/2 -> EXCITATION/3  "<Stator voltage  vq (pu)>"
  EXCITATION/1 -> Vf/1
  Bus Selector/1 -> EXCITATION/2  "<Stator voltage  vd (pu)>"
  Generic Power System Stabilizer/1 -> EXCITATION/4
  Sum2/1 -> Generic Power System Stabilizer/1

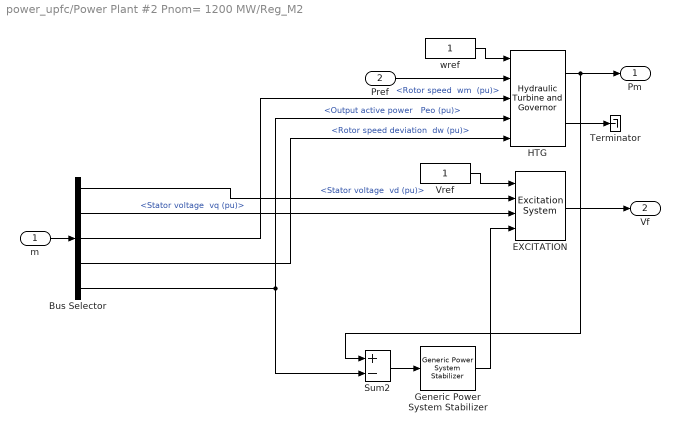
== system power_upfc/Power Plant #2 Pnom= 1200 MW/Reg_M2 ==
  m : Inport
  Pref : Inport  Port=2
  Bus Selector : BusSelector  OutputSignals="dq0 components.Stator voltage  vd (pu),dq0 components.Stator voltage  vq (pu),Mechanical.Rotor speed  wm  (pu),Mechanical.Rotor speed deviation  dw (pu),Output active power   Peo (pu)"
  EXCITATION : sps_avr/Excitation System  tr=20e-3  reg=[ 200, 0.001 ]  exc=[ 1, 0 ]  tgr=[ 0, 0 ]  damp=[ 0.001, 0.1 ]  sat=[ 0, 0 ]  lim="[ 0,  7, 0 ]"  v0=[1,1.41828]
  Generic Power System Stabilizer : powerlib/Machines/Generic Power System Stabilizer  Tsensor=15e-3  K=2.5  Twashout=1  Tleadlag1="[0.06  1]"  Tleadlag2="[0  0]"  VSlimits=[-0.15 0.15]  Vinit=0  Plot_On=off  MagdB_On=on  FreqRange=logspace(-2,2,500)
  HTG : powerlib/Machines/Hydraulic Turbine and Governor  sm="[ 10/3  0.07 ]"  gate="[  0.01  0.97518  -0.1  0.1 ]"  reg="[  0.05  1.163  0.105  0  0.01  ]"  hyd="[  0  2.67  ]"  dref=0  po=0.835333
  Sum2 : Sum  Inputs=+-  SaturateOnIntegerOverflow=on  InputSameDT=on  OutDataTypeStr=Inherit: Same as first input
  Terminator : Terminator
  Vref : Constant
  wref : Constant
  Pm : Outport  InitialOutput=0
  Vf : Outport  Port=2  InitialOutput=0
  wires:
  HTG/2 -> Terminator/1
  Vref/1 -> EXCITATION/1
  m/1 -> Bus Selector/1
  Bus Selector/4 -> HTG/5  "<Rotor speed deviation  dw (pu)>"
  Bus Selector/5 -> HTG/4, Sum2/2  "<Output active power   Peo (pu)>"
  Bus Selector/3 -> HTG/3  "<Rotor speed  wm  (pu)>"
  Pref/1 -> HTG/2
  wref/1 -> HTG/1
  HTG/1 -> Pm/1, Sum2/1
  Bus Selector/2 -> EXCITATION/3  "<Stator voltage  vq (pu)>"
  EXCITATION/1 -> Vf/1
  Bus Selector/1 -> EXCITATION/2  "<Stator voltage  vd (pu)>"
  Generic Power System Stabilizer/1 -> EXCITATION/4
  Sum2/1 -> Generic Power System Stabilizer/1
